simulink model "upper_limit_sliding_mode"  (R2019b)
settings: Solver=VariableStepAuto  StartTime=0.0  StopTime=20  RelTol=1e-3
libraries: fuzblock x1
settings Model: Creator=Alien  LastModifiedBy=Alien
settings SolverCC: ZeroCrossAlgorithm=Adaptive
settings DebuggingCC: IgnoredZcDiagnostic=none

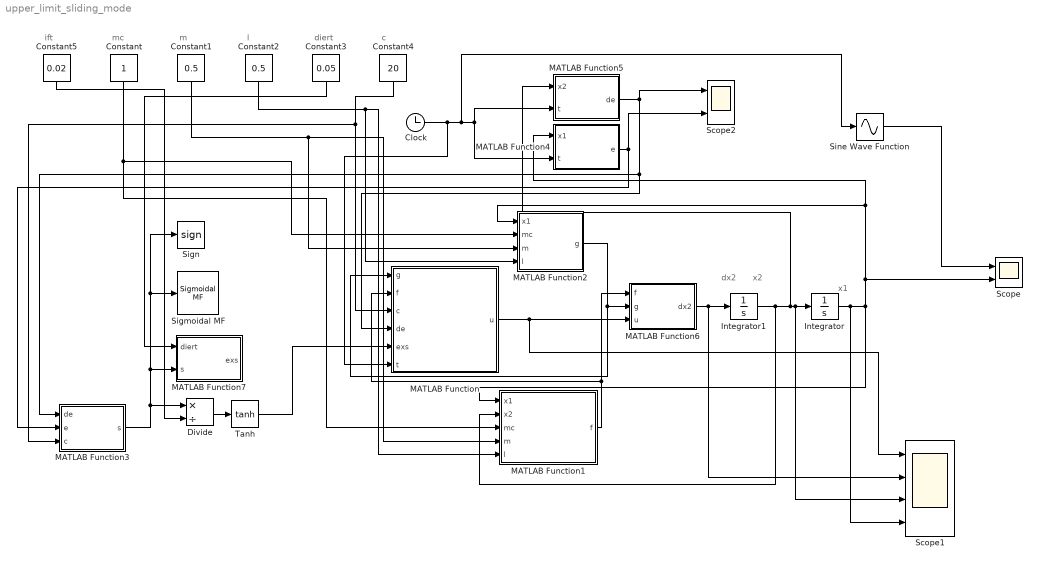
== system upper_limit_sliding_mode ==
  note: c
  note: diert
  note: l
  note: m
  note: mc
  note: dx2
  note: x2
  note: x1
  note: ift
  Clock : Clock
  Constant : Constant
  Constant1 : Constant  Value=0.5
  Constant2 : Constant  Value=0.5
  Constant3 : Constant  Value=0.05
  Constant4 : Constant  Value=20
  Constant5 : Constant  Value=0.02
  Divide : Product  Inputs=*/
  Integrator : Integrator
  Integrator1 : Integrator  InitialCondition=pi/60
  MATLAB Function : MATLAB Function  TreatAsAtomicUnit=on
  MATLAB Function1 : MATLAB Function  TreatAsAtomicUnit=on
  MATLAB Function2 : MATLAB Function  TreatAsAtomicUnit=on
  MATLAB Function3 : MATLAB Function  TreatAsAtomicUnit=on
  MATLAB Function4 : MATLAB Function  TreatAsAtomicUnit=on
  MATLAB Function5 : MATLAB Function  TreatAsAtomicUnit=on
  MATLAB Function6 : MATLAB Function  TreatAsAtomicUnit=on
  MATLAB Function7 : MATLAB Function  TreatAsAtomicUnit=on
  Scope : Scope  NumInputPorts=2
  Scope1 : Scope  NumInputPorts=4
  Scope2 : Scope  NumInputPorts=2
  Sigmoidal MF : fuzblock/Membership  Functions/Sigmoidal MF  a=1  c=0
      settings: SourceProductName=Fuzzy Logic Toolbox  SourceProductBaseCode=FL
  Sign : Signum
  Sine Wave Function : Sin  TimeSource=Use external signal  Amplitude=0.1  SampleTime=0
  Tanh : Trigonometry  Operator=tanh
  wires:
  Integrator1/1 -> MATLAB Function1/2(x2), MATLAB Function5/1(x2), Scope1/3, Integrator/1
  MATLAB Function6/1(dx2) -> Scope1/2, Integrator1/1
  MATLAB Function/1(u) -> Scope1/1, MATLAB Function6/3(u)
  MATLAB Function2/1(g) -> MATLAB Function/1(g), MATLAB Function6/2(g)
  MATLAB Function1/1(f) -> MATLAB Function6/1(f), MATLAB Function/2(f)
  MATLAB Function5/1(de) -> Scope2/1, MATLAB Function3/1(de), MATLAB Function/4(de)
  Integrator/1 -> Scope1/4, MATLAB Function1/1(x1), Scope/2, MATLAB Function4/1(x1), MATLAB Function2/1(x1)
  Constant/1 -> MATLAB Function2/2(mc), MATLAB Function1/3(mc)
  Constant1/1 -> MATLAB Function2/3(m), MATLAB Function1/4(m)
  Constant2/1 -> MATLAB Function2/4(l), MATLAB Function1/5(l)
  MATLAB Function4/1(e) -> Scope2/2, MATLAB Function3/2(e)
  Constant4/1 -> MATLAB Function3/3(c), MATLAB Function/3(c)
  Clock/1 -> MATLAB Function/6(t), Sine Wave Function/1, MATLAB Function4/2(t), MATLAB Function5/2(t)
  MATLAB Function3/1(s) -> MATLAB Function7/2(s), Sign/1, Sigmoidal MF/1, Divide/1
  Sine Wave Function/1 -> Scope/1
  Constant3/1 -> MATLAB Function7/1(diert)
  Divide/1 -> Tanh/1
  Constant5/1 -> Divide/2
  Tanh/1 -> MATLAB Function/5(exs)

== matlab function upper_limit_sliding_mode/MATLAB Function1 ==
  data: x1 input; f output; x2 input; mc input; m input; l input
function f = fcn(x1, x2, mc, m, l)
g = 9.8;
f = (g*sin(x1) - m*l*((x2)^2)*cos(x1)*sin(x1)/(mc +m))/(l*(4/3 - m * ((cos(x1))^2)/(mc + m)));

== matlab function upper_limit_sliding_mode/MATLAB Function ==
  data: g input; u output; f input; c input; de input; exs input; t input
function u = fcn(g, f, c, de, exs, t)
nta = 0.2;
ddx1d = -0.1 * sin(t);
u = 1/g*(ddx1d - f + c * de + nta * exs);

== matlab function upper_limit_sliding_mode/MATLAB Function2 ==
  data: x1 input; g output; mc input; m input; l input
function g = fcn(x1, mc, m, l)
g = (cos(x1)/(mc + m))/(l*(4/3 - m*((cos(x1))^2)/(mc +m)));

== matlab function upper_limit_sliding_mode/MATLAB Function3 ==
  data: de input; s output; e input; c input
function s = fcn(de, e, c)
s = de + c*e;

== matlab function upper_limit_sliding_mode/MATLAB Function4 ==
  data: x1 input; e output; t input
function e = fcn(x1, t)
e = 0.1*sin(t) - x1;

== matlab function upper_limit_sliding_mode/MATLAB Function5 ==
  data: x2 input; de output; t input
function de = fcn(x2, t)
de = 0.1*cos(t) - x2;

== matlab function upper_limit_sliding_mode/MATLAB Function6 ==
  data: f input; g input; u input; dx2 output
function dx2 = fcn(f, g, u)
dx2 = f + g*u;

== matlab function upper_limit_sliding_mode/MATLAB Function7 ==
  data: diert input; exs output; s input
function exs = fcn(diert, s)
if s > diert
    exs = 1;
elseif s < -diert
    exs = -1;
else
    exs = 1/diert*s;
end
